simulink model "adapt2"  (Simulink 6.0)
settings: Solver=ode45  StartTime=0.0  StopTime=10.0  RelTol=1e-3
libraries: dspwin32 x2, dsparch4 x1, dspsrcs4 x1, dspsigops x1, dspadpt3 x1, simulink x1, dspsnks4 x1
settings Model: LastModifiedBy=cclarke  SignalLoggingName=logsOut  BooleanDataType=on  ZeroCrossControl=UseLocalSettings  ProdHWDeviceType=Microprocessor  TargetHWChar=2  TargetHWWordLengths=8,16,32,32  RTWMathFcnLibMatFile=iso_c_tmw.mat  RTWOptions="-aEnforceIntegerDowncast=1 -aFoldNonRolledExpr=1 -aInlineInvariantSignals=1 -aInlineParameters=0 -aLocalBlockOutputs=1 -aRollThreshold=5 -aGenerateReport=0 -aGenCodeOnly=0 -aRTWVerbose=1 -aForceParamTrailComments=0 -aGenerateComments=1 -aIgnoreCustomStorageClasses=1 -aIncHierarchyInIds=0 -aMaxRTWIdLen=31 -aShowEliminatedStatements=0 -aPrefixModelToSubsysFcnNames=1 -aIncDataTypeInIds=0 -aInlinedPrmAccess=\"Literals\" -aTargetFcnLib=\"iso_c_tmw.mat\" -aGenerateFullHeader=1 -aIsPILTarget=0 -aExtMode=0 -aExtModeStaticAlloc=0 -aExtModeTesting=0 -aExtModeStaticAllocSize=1000000 -aExtModeTransport=0 -aLogVarNameModifier=\"rt_\" -aRTWCAPISignals=0 -aRTWCAPIParams=0"
settings DataIOCC: SignalLoggingName=logsOut
settings OptimizationCC: MultiInstanced=off
settings FormatCC: IgnoreBidirectionalLines=off
settings HardwareCC: ProdHWDeviceType=Microprocessor  ShiftRightIntArith=on  TargetHWCharacteristics=InheritFromRTWHook
settings CodeAppCC: FileBanners=off
settings GRTTargetCC: TargetFcnLib=iso_c_tmw.mat  IsERTTarget=off

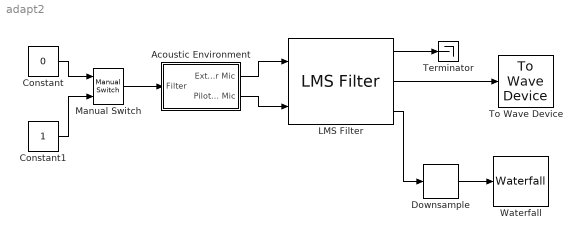
== system adapt2 ==
  Acoustic Environment : Subsystem
  Constant : Constant  Value=0
  Constant1 : Constant
  Downsample : dspsigops/Downsample  N=32  phase=0  ic=0  smode=Allow multirate  fmode=Maintain input frame size
  LMS Filter : dspadpt3/LMS Filter  Algo=Normalized LMS  L=40  stepflag=Dialog  mu=0.002  leakage=1.0  addnparflag=off  ic=0  Adapt=off  resetflag=None  weights=on
  Manual Switch : simulink/Signal Routing/Manual Switch  sw=1  action=0
  Terminator : Terminator
  To Wave Device : dspwin32/To Wave Device  bufDuration=0.4  initDelay=0.05  useDefaultDevice=on  userDeviceID=SoundMAX Digital Audio  enable24Bit=off
  Waterfall : dspsnks4/Waterfall  TraceProperties=off  NumTraces=6  CMapStr=autumn  TNewest=1  TOldest=0  HistoryLength=50  HistoryFull=Overwrite  UpdateInterval=1  ExportMode=All visible  MLExportName=ExportData  AutoExport=off  DisplayProperties=off  MouseMode=Orbit  AxisGrid=on  Snapshot=off  Suspend=off  SyncSnapshots=off  OpenScopeAtSimStart=on  FigPos=[243 195 405 320]  CameraView=[69.4600750684385 564.426060114276 -133.474523953492 0 18.5 3.5 0.616338299486424 -7.9078811427274 1.98411164834144 2.40985953613679 1 18.5 3]  InportDimsHint=[32 1]  AxisProperties=off  AxisColor='w'  XLabel=Amplitude  YLabel=Samples  ZLabel=Time  TriggerProperties=off  TrigStartMode=Immediately  TrigStartT=0  TrigStartN=0  TrigStartFcn=trigbegin  TrigStopMode=Never  TrigStopT=0.1  TrigStopN=1  TrigStopFcn=trigend  TrigRearmMode=Never  TrigRearmT=0  TrigRearmN=0  TrigRearmFcn=trigrearm  XformProperties=on  XformMode=None  XformFcn=abs  XformExpr=(u+1)/2
      settings: YMin=-0.188  YMax=0.179
  wires:
  Constant/1 -> Manual Switch/1
  Manual Switch/1 -> Acoustic Environment/1(Filter)
  Acoustic Environment/1(Exterior Mic) -> LMS Filter/1
  Acoustic Environment/2(Pilot's Mic) -> LMS Filter/2
  Constant1/1 -> Manual Switch/2
  LMS Filter/1 -> Terminator/1
  LMS Filter/2 -> To Wave Device/1
  LMS Filter/3 -> Downsample/1
  Downsample/1 -> Waterfall/1

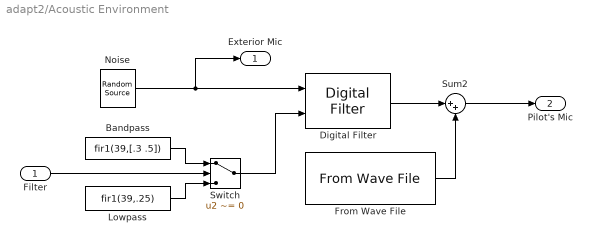
== system adapt2/Acoustic Environment ==
  Filter : Inport
  Bandpass : Constant  Value=fir1(39,[.3 .5])  ShowAdditionalParam=on
  Digital Filter : dsparch4/Digital Filter  TypePopup=FIR (all zeros)  IIRFiltStruct=Direct form II transposed  AllPoleFiltStruct=Direct form  FIRFiltStruct=Direct form  CoeffSource=Input port(s)  NumCoeffs=[1 2]  DenCoeffs=[1 0.1]  BiQuadCoeffs=[1 0.3 0.4 1 0.1 0.2]  LatticeCoeffs=[0.2 0.4]  denIgnore=on  FiltPerSampPopup=One filter per frame  IC=0  ICnum=0  ICden=0  roundingMode=Floor  overflowMode=off
  From Wave File : dspwin32/From Wave File  FileName=dspafxf_8000  SamplesPerFrame=32  MinBufSize=1024  dType=Single  bLoop=on  timesToPlay=inf  restartMode=immediately after last sample  firstSampleOutput=off  lastSampleOutput=off
  Lowpass : Constant  Value=fir1(39,.25)  ShowAdditionalParam=on
  Noise : dspsrcs4/Random Source  SrcType=Gaussian  NormMethod=Sum of uniform values  CltLength=5  Min=-1  Max=1  Mean=0  Var=1  RepMode=Specify seed  Seed=[23341]  Inherit=off  SampMode=Discrete  SampTime=1/8000  SampFrame=32  DataType=Single  OutComplex=Real
  Sum2 : Sum  Inputs=|++  SaturateOnIntegerOverflow=on  InputSameDT=on
  Switch : Switch  Criteria=u2 ~= 0  SaturateOnIntegerOverflow=on
  Exterior Mic : Outport
  Pilot's Mic : Outport  Port=2
  wires:
  From Wave File/1 -> Sum2/2
  Sum2/1 -> Pilot's Mic/1
  Filter/1 -> Switch/2
  Digital Filter/1 -> Sum2/1
  Noise/1 -> Digital Filter/1, Exterior Mic/1
  Switch/1 -> Digital Filter/2
  Bandpass/1 -> Switch/1
  Lowpass/1 -> Switch/3
